simulink model "uav_full_control"  (R2023a)
settings: Solver=FixedStepAuto  StartTime=0.0  StopTime=20  FixedStep=1e-3
undefined symbols (not defined in the file or in its folder): b, c_1, c_2, c_3, c_4, c_5, c_6, c_7, c_8, c_psi, C_SMC, c_z, d, D_rot, D_transl, eps1, eps2, eps3, eps4, eta1, eta2, eta3, eta4, eulerlimit, g, J1, J2, J3, Jr, K, k1, k2, k3, K_lqr, k_phi, K_SMC, k_theta, L, m, Matrix_Force2angular_velocity, R
libraries: simulink x14, control_form_LagrangeSimplified x2, control_form_NL x2, control_form_NL_forces x2, control_form_LagrangeSimplified_forces x1
(part 2 of 2)

== matlab function uav_full_control/MATLAB Function5 ==
  data: x input; transf output; y input; z input; phi input; theta input; psi input; xdot input; ydot input; zdot input; zeta input; xi input; p input; q input; r input
function transf = transform_difeo_function(x,y,z,phi,theta,psi,xdot,ydot,zdot,zeta,xi,p,q,r)

% prep
m=1.88;
g=9.81;
J1=1.453e-2;
J2=1.453e-2;
J3=2.884e-2;

input1=0;
input2=0;
input3=0;
input4=0;

sphi=sin(phi);
cphi=cos(phi);
stheta=sin(theta);
ctheta=cos(theta);
spsi=sin(psi);
cpsi=cos(psi);

% model dynamics
phi_dot=p+q*(sin(phi)*tan(theta))+r*(cos(phi)*tan(theta));
theta_dot=q*cos(phi)-r*sin(phi);
psi_dot=q*sin(phi)/cos(theta)+r*cos(phi)/cos(theta);


zeta_dot=xi;
xi_dot=input1;

p_dot=(J2-J3)/J1*q*r+1/J1*input2;
q_dot=(J3-J1)/J2*r*p+1/J2*input3;
r_dot=(J1-J2)/J3*p*q+1/J3*input4;

%others
phi_d_dot=p_dot+q_dot*sphi*tan(theta)+phi_dot*q*cphi*tan(theta)+theta_dot*q*sphi/(ctheta^2)+...
r_dot*cphi*tan(theta)-phi_dot*r*sphi*tan(theta)+theta_dot*r*cphi/(ctheta^2);

theta_d_dot=q_dot*cphi-phi_dot*q*sphi-r_dot*sphi-r*phi_dot*cphi;

psi_d_dot=q_dot*sphi/ctheta+q/(ctheta^2)*(phi_dot*cphi*ctheta+theta_dot*sphi*stheta)+...
r_dot*cphi/ctheta+r/(ctheta^2)*(-phi_dot*sphi*ctheta+theta_dot*cphi*stheta);

%%%--------------------------------------------------------------------------------------

%x

Cx=cphi*stheta*cpsi+sphi*spsi;

Cx_dot=-phi_dot*sphi*stheta*cpsi+theta_dot*cphi*ctheta*cpsi-psi_dot*cphi*stheta*spsi...
+phi_dot*cphi*spsi+psi_dot*sphi*cpsi;

Cx_d_dot=psi_d_dot*(-sphi*stheta*cpsi+cphi*spsi)+theta_d_dot*cphi*ctheta*cpsi...
+psi_d_dot*(-cphi*stheta*spsi+sphi*cpsi)-cphi*stheta*cpsi*(phi_dot^2+theta_dot^2+psi_dot^2)...
-2*phi_dot*theta_dot*sphi*ctheta*cpsi+2*phi_dot*psi_dot*sphi*stheta*spsi...
-2*theta_dot*psi_dot*cphi*ctheta*spsi-sphi*spsi*(phi_dot^2+psi_dot^2)+2*phi_dot*psi_dot*cphi*cpsi;

x_4dots=-1/m*(input1*Cx+2*xi*Cx_dot+zeta*Cx_d_dot); % Lf4h1(x)
LgLf3h1=-1/m*[Cx,...
    1/J1*zeta*(-sphi*stheta*cpsi+cphi*spsi),...
    1/J2*zeta*((-sphi*stheta*cpsi+cphi*spsi)*sphi*tan(theta)+cphi*ctheta*cpsi*cphi+...
    (-cphi*stheta*spsi+sphi*cpsi)*sphi/ctheta),...
    1/J3*zeta*((-sphi*stheta*cpsi+cphi*spsi)*cphi*tan(theta)-cphi*ctheta*cpsi*sphi+...
    (-cphi*stheta*spsi+sphi*cpsi)*cphi/ctheta)];

Lf0h1=x;
Lf1h1=xdot;
Lf2h1=-1/m*zeta*Cx;
Lf3h1=-1/m*(xi*Cx+zeta*Cx_dot);

%y

Cy=cphi*stheta*spsi-sphi*cpsi;

Cy_dot=-phi_dot*sphi*stheta*spsi+theta_dot*cphi*ctheta*spsi+psi_dot*cphi*stheta*cpsi...
-phi_dot*cphi*cpsi+psi_dot*sphi*spsi;

Cy_d_dot=phi_d_dot*(-sphi*stheta*spsi-cphi*cpsi)+theta_d_dot*cphi*ctheta*spsi...
+psi_d_dot*(cphi*stheta*cpsi+sphi*spsi)-cphi*stheta*spsi*(phi_dot^2+theta_dot^2+psi_dot^2)...
-2*phi_dot*theta_dot*sphi*ctheta*spsi-2*phi_dot*psi_dot*sphi*stheta*cpsi...
+2*theta_dot*psi_dot*cphi*ctheta*cpsi+sphi*cpsi*(phi_dot^2+psi_dot^2)+2*phi_dot*psi_dot*cphi*spsi;

y_4dots=-1/m*(input1*Cy+2*xi*Cy_dot+zeta*Cy_d_dot);
LgLf3h2=-1/m*[Cy,...
    1/J1*zeta*(-sphi*stheta*spsi-cphi*cpsi),...
    1/J2*zeta*((-sphi*stheta*spsi-cphi*cpsi)*sphi*tan(theta)+cphi*ctheta*spsi*cphi+...
    (cphi*stheta*cpsi+sphi*spsi)*sphi/ctheta),...
    1/J3*zeta*((-sphi*stheta*spsi-cphi*cpsi)*cphi*tan(theta)-cphi*ctheta*spsi*sphi+...
    (cphi*stheta*cpsi+sphi*spsi)*cphi/ctheta)];

Lf0h2=y;
Lf1h2=ydot;
Lf2h2=-1/m*zeta*Cy;
Lf3h2=-1/m*(xi*Cy+zeta*Cy_dot);

%z
Cz=cphi*ctheta;

Cz_dot=-phi_dot*sphi*ctheta-theta_dot*cphi*stheta;

Cz_d_dot=-phi_d_dot*sphi*ctheta-phi_dot^2*cphi*ctheta+2*phi_dot*theta_dot*sphi*stheta...
    -theta_d_dot*cphi*stheta-theta_dot^2*cphi*ctheta;

z_4dots=-1/m*(input1*Cz+2*xi*Cz_dot+zeta*Cz_d_dot);
LgLf3h3=-1/m*[Cz,...
    1/J1*zeta*(-sphi*ctheta),...
    1/J2*zeta*(-sphi*ctheta*sphi*tan(theta)-cphi*stheta*cphi),...
    1/J3*zeta*(-sphi*ctheta*cphi*tan(theta)+cphi*stheta*sphi)];

Lf0h3=z;
Lf1h3=zdot;
Lf2h3=g-1/m*zeta*Cz;
Lf3h3=-1/m*(xi*Cz+zeta*Cz_dot);
%psi
Lf0h4=psi;
Lf1h4=psi_dot;
%psi_d_dot is defined above
LgLf1h4=[0,...
    0,...
    1/J2*sphi/ctheta,...
    1/J3*cphi/ctheta];
transf=[Lf0h1,Lf1h1,Lf2h1,Lf3h1,Lf0h2,Lf1h2,Lf2h2,Lf3h2,Lf0h3,Lf1h3,Lf2h3,Lf3h3,Lf0h4,Lf1h4]';

== matlab function uav_full_control/MATLAB Function6 ==
  data: states input; v_hat input; fr_hat input; C_SMC input; k_theta input; k_phi input; K_SMC input; xref input; yref input; zref input; psiref input; u output
function u = fcn_smc(states, v_hat, fr_hat, C_SMC, k_theta, k_phi, K_SMC, xref, yref, zref, psiref)
    arguments
        states (12,1) {mustBeNumeric}
        v_hat
        fr_hat
        C_SMC 
        k_theta
        k_phi
        K_SMC
        xref (5,1)
        yref (5,1)
        zref (5,1)
        psiref (3,1)
    end

 m=1.888;
 g=9.81;
 J1=1.453e-2;
 J2=1.453e-2;
 J3=2.884e-2;

 x=states(1);
 y=states(2);
 z=states(3);
 phi=states(4);
 theta=states(5);
 psi=states(6);
 xdot=states(7);
 ydot=states(8);
 zdot=states(9);
 phidot=states(10);
 thetadot=states(11);
 psidot=states(12);

 xdesired=xref(1);
 xdesired_dot=xref(2);
 ydesired=yref(1);
 ydesired_dot=yref(2);
 zdesired=zref(1);
 zdesired_dot=zref(2);
 psidesired=psiref(1);
 psidesired_dot=psiref(2);
 xdesired_d_dot=xref(3);
 ydesired_d_dot=yref(3);
 zdesired_d_dot=zref(3);
 psidesired_d_dot=psiref(3);


 ex=x-xdesired;
 ex_dot=xdot-xdesired_dot;
 ey=y-ydesired;
 ey_dot=ydot-ydesired_dot;
 ez=z-zdesired;
 ez_dot=zdot-zdesired_dot;
 epsi=psi-psidesired;
 epsi_dot=psidot-psidesired_dot;
 
 % x_d_dot=-1/m*(cos(phi)*sin(theta)*cos(psi)+sin(phi)*sin(psi))*u1; 
 % y_d_dot=-1/m*(cos(phi)*sin(theta)*sin(psi)-sin(phi)*cos(psi))*u1;
 % 
 % x_dots_3=-1/m*(-phidot*sin(phi)*sin(theta)*cos(psi)+thetadot*cos(phi)*cos(theta)*cos(psi)-...
 %     psidot*cos(phi)*sin(theta)*sin(psi)+phidot*cos(phi)*sin(psi)+psidot*sin(phi)*cos(psi))*u1+u1dot*-1/m*(cos(phi)*sin(theta)*cos(psi)+sin(phi)*sin(psi));
 % y_dots_3=-1/m*(-phidot*sin(phi)*sin(theta)*sin(psi)+thetadot*cos(phi)*cos(theta)*sin(psi)+...
 %     psidot*cos(phi)*sin(theta)*cos(psi)-phidot*cos(phi)*cos(psi)+psidot*sin(phi)*sin(psi))*u1+u1dot*-1/m*(cos(phi)*sin(theta)*sin(psi)-sin(phi)*cos(psi));

 x_d_dot=-1/m*(cos(phi)*sin(theta)*cos(psi)+sin(phi)*sin(psi)); 
 y_d_dot=-1/m*(cos(phi)*sin(theta)*sin(psi)-sin(phi)*cos(psi));

 x_dots_3=-1/m*(-phidot*sin(phi)*sin(theta)*cos(psi)+thetadot*cos(phi)*cos(theta)*cos(psi)-...
     psidot*cos(phi)*sin(theta)*sin(psi)+phidot*cos(phi)*sin(psi)+psidot*sin(phi)*cos(psi));
 y_dots_3=-1/m*(-phidot*sin(phi)*sin(theta)*sin(psi)+thetadot*cos(phi)*cos(theta)*sin(psi)+...
     psidot*cos(phi)*sin(theta)*cos(psi)-phidot*cos(phi)*cos(psi)+psidot*sin(phi)*sin(psi));

 thetadesired=ex_dot+k_theta*ex;
 thetadesired_dot=(x_d_dot-xref(3))+k_theta*ex_dot;
 phidesired=ey_dot+k_phi*ey;
 phidesired_dot=(y_d_dot-yref(3))+k_phi*ey_dot;

 thetadesired_d_dot=(x_dots_3-xref(4))+k_theta*(x_d_dot-xdesired_d_dot);
 phidesired_d_dot=(y_dots_3-yref(4))+k_phi*(y_d_dot-ydesired_d_dot);
 %

 
 ephi=phi-phidesired;
 ephi_dot=phidot-phidesired_dot;
 etheta=theta-thetadesired;
 etheta_dot=thetadot-thetadesired_dot;

 e=[ex ey ez ephi etheta epsi]';
 e_dot=[ex_dot ey_dot ez_dot ephi_dot etheta_dot epsi_dot]';
 
 s=e_dot+K_SMC*e;

 G=[x_d_dot,0,0,0,1,0;...
     y_d_dot,0,0,0,0,1;
     -1/m*cos(phi)*cos(theta),0,0,0,0,0;
     0,1/J1,0,0,0,0;
     0,0,1/J2,0,0,0;
     0,0,0,1/J3,0,0];
 Ginv=inv(G);

 f=[0;0;g;(J2-J3)/J1*thetadot*psidot;(J3-J1)/J2*psidot*phidot;(J1-J2)/J3*phidot*thetadot];
 state_desired_d_dot=[xdesired_d_dot ydesired_d_dot zdesired_d_dot phidesired_d_dot thetadesired_d_dot psidesired_d_dot]';
% u=Ginv*(-f+v_hat-fr_hat+state_desired_d_dot-K_SMC*e_dot-diag([C_SMC(1),C_SMC(2),C_SMC(3),C_SMC(4),C_SMC(5),C_SMC(6)])*[sign(s(1)) sign(s(2)) sign(s(3)) sign(s(4)) sign(s(5)) sign(s(6))]');
u=Ginv*(-f+v_hat-fr_hat+state_desired_d_dot-K_SMC*e_dot-diag([C_SMC(1),C_SMC(2),C_SMC(3),C_SMC(4),C_SMC(5),C_SMC(6)])*[saturation_f(s(1)/0.3) saturation_f(s(2)/0.3) saturation_f(s(3)/0.3) saturation_f(s(4)/0.3) saturation_f(s(5)/0.3) saturation_f(s(6)/0.3)]');
% u=Ginv*(-f-fr_hat+state_desired_d_dot-K_SMC*e_dot-diag([C_SMC(1),C_SMC(2),C_SMC(3),C_SMC(4),C_SMC(5),C_SMC(6)])*[sign(s(1)) sign(s(2)) sign(s(3)) sign(s(4)) sign(s(5)) sign(s(6))]');


 function out=saturation_f(x) 
    if(abs(x)<=1)
        out=x;
    else
        out=x/abs(x);
    end
end
end

== matlab function uav_full_control/u1 ==
  data: states input; c_z input; eps1 input; eta1 input; u1 output; zref input
function u1 = fcn_u1(states, c_z,eps1,eta1,zref)
    arguments
        states (12,1) {mustBeNumeric}
        c_z
        eps1
        eta1
        zref (5,1) {mustBeNumeric}
    end

 m=1.888;
 g=9.81;
 J1=1.453e-2;
 J2=1.453e-2;
 J3=2.884e-2;

 x=states(1);
 y=states(2);
 z=states(3);
 phi=states(4);
 theta=states(5);
 psi=states(6);
 xdot=states(7);
 ydot=states(8);
 zdot=states(9);
 phidot=states(10);
 thetadot=states(11);
 psidot=states(12);

 zdesired=zref(1);
 zdesired_dot=zref(2);
 zdesired_d_dot=zref(3);
 
 s1=c_z*(zdesired-z)+zdesired_dot-zdot;
 u1=m/(cos(phi)*cos(theta))*(g-zdesired_d_dot-c_z*(zdesired_dot-zdot)-eps1*saturation_f(s1/0.3)-eta1*s1);

  function out=saturation_f(x) 
    if(abs(x)<=1)
        out=x;
    else
        out=x/abs(x);
    end
end
end

== matlab function uav_full_control/u2 ==
  data: states input; c_5 input; c_6 input; c_7 input; u2 output; c_8 input; eps4 input; eta4 input; c_z input; eps1 input; eta1 input; zref input; yref input; phiref input
function u2 = fcn_u2(states, c_5,c_6,c_7,c_8,eps4,eta4, c_z, eps1, eta1, zref,yref,phiref)
    arguments
        states (12,1) {mustBeNumeric}
        c_5
        c_6
        c_7
        c_8
        eps4
        eta4
        c_z
        eps1
        eta1
        zref 
        yref (5,1) {mustBeNumeric}
        phiref (3,1) {mustBeNumeric}
    end

 m=1.888;
 g=9.81;
 J1=1.453e-2;
 J2=1.453e-2;
 J3=2.884e-2;
 D_rot=diag([0.3,0.3,0.1]);

 x=states(1);
 y=states(2);
 z=states(3);
 phi=states(4);
 theta=states(5);
 psi=states(6);
 xdot=states(7);
 ydot=states(8);
 zdot=states(9);
 phidot=states(10);
 thetadot=states(11);
 psidot=states(12);
 
  %u1
 zdesired=zref(1);
 zdesired_dot=zref(2);
 zdesired_d_dot=zref(3);
 
 s1=c_z*(zdesired-z)+zdesired_dot-zdot;
 u1=m/(cos(phi)*cos(theta))*(g-zdesired_d_dot-c_z*(zdesired_dot-zdot)-eps1*saturation_f(s1/0.3)-eta1*s1);

  %u2
  ydesired=yref(1);
  ydesired_dot=yref(2);
  ydesired_d_dot=yref(3);
  phidesired=phiref(1);
  phidesired_dot=phiref(2);
  phidesired_d_dot=phiref(3);
  y_d_dot=-1/m*(cos(phi)*sin(theta)*sin(psi)-sin(phi)*cos(psi))*u1;
 
 c_5=c_5/(u1*cos(psi));
 c_6=c_6/(u1*cos(psi));

 s4=c_5*(ydesired_dot-ydot)+c_6*(ydesired-y)+c_7*(phidesired_dot-phidot)+c_8*(phidesired-phi);
 u2=J1/c_7*(phidesired_d_dot+D_rot(1,1)*phidot/J1-(J2-J3)/J1*thetadot*psidot+c_8*(phidesired_dot-phidot)+c_6*(ydesired_dot-ydot)+c_5*(ydesired_d_dot-y_d_dot)+eps4*saturation_f(s4/0.3)+eta4*s4);

 function out=saturation_f(x) 
    if(abs(x)<=1)
        out=x;
    else
        out=x/abs(x);
    end
 end
end

== matlab function uav_full_control/u3 ==
  data: states input; c_1 input; c_2 input; c_3 input; u3 output; c_4 input; eps3 input; eta3 input; c_z input; eps1 input; eta1 input; zref input; xref input; thetaref input
function u3 = fcn_u3(states, c_1,c_2,c_3,c_4,eps3,eta3,c_z, eps1, eta1, zref,xref,thetaref)
    arguments
        states (12,1) {mustBeNumeric}
        c_1
        c_2
        c_3
        c_4
        eps3
        eta3
        c_z
        eps1
        eta1
        zref
        xref (5,1) {mustBeNumeric}
        thetaref (3,1) {mustBeNumeric}
    end

 m=1.888;
 g=9.81;
 J1=1.453e-2;
 J2=1.453e-2;
 J3=2.884e-2;
 D_rot=diag([0.3,0.3,0.1]);


 x=states(1);
 y=states(2);
 z=states(3);
 phi=states(4);
 theta=states(5);
 psi=states(6);
 xdot=states(7);
 ydot=states(8);
 zdot=states(9);
 phidot=states(10);
 thetadot=states(11);
 psidot=states(12);

 %u1
 zdesired=zref(1);
 zdesired_dot=zref(2);
 zdesired_d_dot=zref(3);
 
 s1=c_z*(zdesired-z)+zdesired_dot-zdot;
 u1=m/(cos(phi)*cos(theta))*(g-zdesired_d_dot-c_z*(zdesired_dot-zdot)-eps1*saturation_f(s1/0.3)-eta1*s1);
 
 %u3
 xdesired=xref(1);
 xdesired_dot=xref(2);
 xdesired_d_dot=xref(3);
 thetadesired=thetaref(1);
 thetadesired_dot=thetaref(2);
 thetadesired_d_dot=thetaref(3);
 x_d_dot=-1/m*(cos(phi)*sin(theta)*cos(psi)+sin(phi)*sin(psi))*u1;

 c_1=c_1/(u1*cos(phi)*cos(psi));
 c_2=c_2/(u1*cos(phi)*cos(psi));

 s3=c_1*(xdesired_dot-xdot)+c_2*(xdesired-x)+c_3*(thetadesired_dot-thetadot)+c_4*(thetadesired-theta);
 u3=J2/c_3*(thetadesired_d_dot+D_rot(2,2)*thetadot/J2-(J3-J1)/J2*psidot*phidot+c_4*(thetadesired_dot-thetadot)+c_2*(xdesired_dot-xdot)+c_1*(xdesired_d_dot-x_d_dot)+eps3*saturation_f(s3/0.3)+eta3*s3);
 function out=saturation_f(x) 
    if(abs(x)<=1)
        out=x;
    else
        out=x/abs(x);
    end
end
end

== matlab function uav_full_control/u4 ==
  data: states input; c_psi input; eps2 input; eta2 input; u4 output; psiref input
function u4 = fcn_u4(states, c_psi,eps2,eta2,psiref)
    arguments
        states (12,1) {mustBeNumeric}
        c_psi
        eps2
        eta2
        psiref (3,1) {mustBeNumeric}
    end

 m=1.888;
 g=9.81;
 J1=1.453e-2;
 J2=1.453e-2;
 J3=2.884e-2;

 x=states(1);
 y=states(2);
 z=states(3);
 phi=states(4);
 theta=states(5);
 psi=states(6);
 xdot=states(7);
 ydot=states(8);
 zdot=states(9);
 phidot=states(10);
 thetadot=states(11);
 psidot=states(12);

 psidesired=psiref(1);
 psidesired_dot=psiref(2);
 psidesired_d_dot=psiref(3);
 
 s2=c_psi*(psidesired-psi)+psidesired_dot-psidot;
 u4=J3*(psidesired_d_dot-(J1-J2)/J3*phidot*thetadot+c_psi*(psidesired_dot-psidot)+eps2*sign(s2)+eta2*s2);
end

== matlab function uav_full_control/MATLAB Function1 ==
  data: x input; b output; y input; z input; phi input; theta input; psi input; xdot input; ydot input; zdot input; zeta input; xi input; p input; q input; r input
function b = b_function(x,y,z,phi,theta,psi,xdot,ydot,zdot,zeta,xi,p,q,r)

% prep
m=1.88;
g=9.81;
J1=1.453e-2;
J2=1.453e-2;
J3=2.884e-2;

input1=0;
input2=0;
input3=0;
input4=0;

sphi=sin(phi);
cphi=cos(phi);
stheta=sin(theta);
ctheta=cos(theta);
spsi=sin(psi);
cpsi=cos(psi);

% model dynamics
phi_dot=p+q*(sin(phi)*tan(theta))+r*(cos(phi)*tan(theta));
theta_dot=q*cos(phi)-r*sin(phi);
psi_dot=q*sin(phi)/cos(theta)+r*cos(phi)/cos(theta);


zeta_dot=xi;
xi_dot=input1;

p_dot=(J2-J3)/J1*q*r+1/J1*input2;
q_dot=(J3-J1)/J2*r*p+1/J2*input3;
r_dot=(J1-J2)/J3*p*q+1/J3*input4;

%others
phi_d_dot=p_dot+q_dot*sphi*tan(theta)+phi_dot*q*cphi*tan(theta)+theta_dot*q*sphi/(ctheta^2)+...
r_dot*cphi*tan(theta)-phi_dot*r*sphi*tan(theta)+theta_dot*r*cphi/(ctheta^2);

theta_d_dot=q_dot*cphi-phi_dot*q*sphi-r_dot*sphi-r*phi_dot*cphi;

psi_d_dot=q_dot*sphi/ctheta+q/(ctheta^2)*(phi_dot*cphi*ctheta+theta_dot*sphi*stheta)+...
r_dot*cphi/ctheta+r/(ctheta^2)*(-phi_dot*sphi*ctheta+theta_dot*cphi*stheta);

%%%--------------------------------------------------------------------------------------

%x

Cx=cphi*stheta*cpsi+sphi*spsi;

Cx_dot=-phi_dot*sphi*stheta*cpsi+theta_dot*cphi*ctheta*cpsi-psi_dot*cphi*stheta*spsi...
+phi_dot*cphi*spsi+psi_dot*sphi*cpsi;

Cx_d_dot=psi_d_dot*(-sphi*stheta*cpsi+cphi*spsi)+theta_d_dot*cphi*ctheta*cpsi...
+psi_d_dot*(-cphi*stheta*spsi+sphi*cpsi)-cphi*stheta*cpsi*(phi_dot^2+theta_dot^2+psi_dot^2)...
-2*phi_dot*theta_dot*sphi*ctheta*cpsi+2*phi_dot*psi_dot*sphi*stheta*spsi...
-2*theta_dot*psi_dot*cphi*ctheta*spsi-sphi*spsi*(phi_dot^2+psi_dot^2)+2*phi_dot*psi_dot*cphi*cpsi;

x_4dots=-1/m*(input1*Cx+2*xi*Cx_dot+zeta*Cx_d_dot); % Lf4h1(x)
LgLf3h1=-1/m*[Cx,...
    1/J1*zeta*(-sphi*stheta*cpsi+cphi*spsi),...
    1/J2*zeta*((-sphi*stheta*cpsi+cphi*spsi)*sphi*tan(theta)+cphi*ctheta*cpsi*cphi+...
    (-cphi*stheta*spsi+sphi*cpsi)*sphi/ctheta),...
    1/J3*zeta*((-sphi*stheta*cpsi+cphi*spsi)*cphi*tan(theta)-cphi*ctheta*cpsi*sphi+...
    (-cphi*stheta*spsi+sphi*cpsi)*cphi/ctheta)];

%y

Cy=cphi*stheta*spsi-sphi*cpsi;

Cy_dot=-phi_dot*sphi*stheta*spsi+theta_dot*cphi*ctheta*spsi+psi_dot*cphi*stheta*cpsi...
-phi_dot*cphi*cpsi+psi_dot*sphi*spsi;

Cy_d_dot=phi_d_dot*(-sphi*stheta*spsi-cphi*cpsi)+theta_d_dot*cphi*ctheta*spsi...
+psi_d_dot*(cphi*stheta*cpsi+sphi*spsi)-cphi*stheta*spsi*(phi_dot^2+theta_dot^2+psi_dot^2)...
-2*phi_dot*theta_dot*sphi*ctheta*spsi-2*phi_dot*psi_dot*sphi*stheta*cpsi...
+2*theta_dot*psi_dot*cphi*ctheta*cpsi+sphi*cpsi*(phi_dot^2+psi_dot^2)+2*phi_dot*psi_dot*cphi*spsi;

y_4dots=-1/m*(input1*Cy+2*xi*Cy_dot+zeta*Cy_d_dot);
LgLf3h2=-1/m*[Cy,...
    1/J1*zeta*(-sphi*stheta*spsi-cphi*cpsi),...
    1/J2*zeta*((-sphi*stheta*spsi-cphi*cpsi)*sphi*tan(theta)+cphi*ctheta*spsi*cphi+...
    (cphi*stheta*cpsi+sphi*spsi)*sphi/ctheta),...
    1/J3*zeta*((-sphi*stheta*spsi-cphi*cpsi)*cphi*tan(theta)-cphi*ctheta*spsi*sphi+...
    (cphi*stheta*cpsi+sphi*spsi)*cphi/ctheta)];
%z
Cz=cphi*ctheta;

Cz_dot=-phi_dot*sphi*ctheta-theta_dot*cphi*stheta;

Cz_d_dot=-phi_d_dot*sphi*ctheta-phi_dot^2*cphi*ctheta+2*phi_dot*theta_dot*sphi*stheta...
    -theta_d_dot*cphi*stheta-theta_dot^2*cphi*ctheta;

z_4dots=-1/m*(input1*Cz+2*xi*Cz_dot+zeta*Cz_d_dot);
LgLf3h3=-1/m*[Cz,...
    1/J1*zeta*(-sphi*ctheta),...
    1/J2*zeta*(-sphi*ctheta*sphi*tan(theta)-cphi*stheta*cphi),...
    1/J3*zeta*(-sphi*ctheta*cphi*tan(theta)+cphi*stheta*sphi)];

%psi

%psi_d_dot is defined above
LgLf1h4=[0,...
    0,...
    1/J2*sphi/ctheta,...
    1/J3*cphi/ctheta];
b=[x_4dots;y_4dots;z_4dots;psi_d_dot];

== matlab function uav_full_control/MATLAB Function ==
  data: x input; delta_inv output; y input; z input; phi input; theta input; psi input; xdot input; ydot input; zdot input; zeta input; xi input; p input; q input; r input
function delta_inv = delta_inv_function(x,y,z,phi,theta,psi,xdot,ydot,zdot,zeta,xi,p,q,r)

% prep
m=1.88;
g=9.81;
J1=1.453e-2;
J2=1.453e-2;
J3=2.884e-2;

input1=0;
input2=0;
input3=0;
input4=0;

sphi=sin(phi);
cphi=cos(phi);
stheta=sin(theta);
ctheta=cos(theta);
spsi=sin(psi);
cpsi=cos(psi);

% model dynamics
phi_dot=p+q*(sin(phi)*tan(theta))+r*(cos(phi)*tan(theta));
theta_dot=q*cos(phi)-r*sin(phi);
psi_dot=q*sin(phi)/cos(theta)+r*cos(phi)/cos(theta);


zeta_dot=xi;
xi_dot=input1;

p_dot=(J2-J3)/J1*q*r+1/J1*input2;
q_dot=(J3-J1)/J2*r*p+1/J2*input3;
r_dot=(J1-J2)/J3*p*q+1/J3*input4;

%others
phi_d_dot=p_dot+q_dot*sphi*tan(theta)+phi_dot*q*cphi*tan(theta)+theta_dot*q*sphi/(ctheta^2)+...
r_dot*cphi*tan(theta)-phi_dot*r*sphi*tan(theta)+theta_dot*r*cphi/(ctheta^2);

theta_d_dot=q_dot*cphi-phi_dot*q*sphi-r_dot*sphi-r*phi_dot*cphi;

psi_d_dot=q_dot*sphi/ctheta+q/(ctheta^2)*(phi_dot*cphi*ctheta+theta_dot*sphi*stheta)+...
r_dot*cphi/ctheta+r/(ctheta^2)*(-phi_dot*sphi*ctheta+theta_dot*cphi*stheta);

%%%--------------------------------------------------------------------------------------

%x

Cx=cphi*stheta*cpsi+sphi*spsi;

Cx_dot=-phi_dot*sphi*stheta*cpsi+theta_dot*cphi*ctheta*cpsi-psi_dot*cphi*stheta*spsi...
+phi_dot*cphi*spsi+psi_dot*sphi*cpsi;

Cx_d_dot=psi_d_dot*(-sphi*stheta*cpsi+cphi*spsi)+theta_d_dot*cphi*ctheta*cpsi...
+psi_d_dot*(-cphi*stheta*spsi+sphi*cpsi)-cphi*stheta*cpsi*(phi_dot^2+theta_dot^2+psi_dot^2)...
-2*phi_dot*theta_dot*sphi*ctheta*cpsi+2*phi_dot*psi_dot*sphi*stheta*spsi...
-2*theta_dot*psi_dot*cphi*ctheta*spsi-sphi*spsi*(phi_dot^2+psi_dot^2)+2*phi_dot*psi_dot*cphi*cpsi;

x_4dots=-1/m*(input1*Cx+2*xi*Cx_dot+zeta*Cx_d_dot); % Lf4h1(x)
LgLf3h1=-1/m*[Cx,...
    1/J1*zeta*(-sphi*stheta*cpsi+cphi*spsi),...
    1/J2*zeta*((-sphi*stheta*cpsi+cphi*spsi)*sphi*tan(theta)+cphi*ctheta*cpsi*cphi+...
    (-cphi*stheta*spsi+sphi*cpsi)*sphi/ctheta),...
    1/J3*zeta*((-sphi*stheta*cpsi+cphi*spsi)*cphi*tan(theta)-cphi*ctheta*cpsi*sphi+...
    (-cphi*stheta*spsi+sphi*cpsi)*cphi/ctheta)];

%y

Cy=cphi*stheta*spsi-sphi*cpsi;

Cy_dot=-phi_dot*sphi*stheta*spsi+theta_dot*cphi*ctheta*spsi+psi_dot*cphi*stheta*cpsi...
-phi_dot*cphi*cpsi+psi_dot*sphi*spsi;

Cy_d_dot=phi_d_dot*(-sphi*stheta*spsi-cphi*cpsi)+theta_d_dot*cphi*ctheta*spsi...
+psi_d_dot*(cphi*stheta*cpsi+sphi*spsi)-cphi*stheta*spsi*(phi_dot^2+theta_dot^2+psi_dot^2)...
-2*phi_dot*theta_dot*sphi*ctheta*spsi-2*phi_dot*psi_dot*sphi*stheta*cpsi...
+2*theta_dot*psi_dot*cphi*ctheta*cpsi+sphi*cpsi*(phi_dot^2+psi_dot^2)+2*phi_dot*psi_dot*cphi*spsi;

y_4dots=-1/m*(input1*Cy+2*xi*Cy_dot+zeta*Cy_d_dot);
LgLf3h2=-1/m*[Cy,...
    1/J1*zeta*(-sphi*stheta*spsi-cphi*cpsi),...
    1/J2*zeta*((-sphi*stheta*spsi-cphi*cpsi)*sphi*tan(theta)+cphi*ctheta*spsi*cphi+...
    (cphi*stheta*cpsi+sphi*spsi)*sphi/ctheta),...
    1/J3*zeta*((-sphi*stheta*spsi-cphi*cpsi)*cphi*tan(theta)-cphi*ctheta*spsi*sphi+...
    (cphi*stheta*cpsi+sphi*spsi)*cphi/ctheta)];
%z
Cz=cphi*ctheta;

Cz_dot=-phi_dot*sphi*ctheta-theta_dot*cphi*stheta;

Cz_d_dot=-phi_d_dot*sphi*ctheta-phi_dot^2*cphi*ctheta+2*phi_dot*theta_dot*sphi*stheta...
    -theta_d_dot*cphi*stheta-theta_dot^2*cphi*ctheta;

z_4dots=-1/m*(input1*Cz+2*xi*Cz_dot+zeta*Cz_d_dot);
LgLf3h3=-1/m*[Cz,...
    1/J1*zeta*(-sphi*ctheta),...
    1/J2*zeta*(-sphi*ctheta*sphi*tan(theta)-cphi*stheta*cphi),...
    1/J3*zeta*(-sphi*ctheta*cphi*tan(theta)+cphi*stheta*sphi)];

%psi

%psi_d_dot is defined above
LgLf1h4=[0,...
    0,...
    1/J2*sphi/ctheta,...
    1/J3*cphi/ctheta];
delta_inv = inv([LgLf3h1;LgLf3h2;LgLf3h3;LgLf1h4]);

== matlab function uav_full_control/MATLAB Function2 ==
  data: x input; transf output; y input; z input; phi input; theta input; psi input; xdot input; ydot input; zdot input; zeta input; xi input; p input; q input; r input
function transf = transform_difeo_function(x,y,z,phi,theta,psi,xdot,ydot,zdot,zeta,xi,p,q,r)

% prep
m=1.88;
g=9.81;
J1=1.453e-2;
J2=1.453e-2;
J3=2.884e-2;

input1=0;
input2=0;
input3=0;
input4=0;

sphi=sin(phi);
cphi=cos(phi);
stheta=sin(theta);
ctheta=cos(theta);
spsi=sin(psi);
cpsi=cos(psi);

% model dynamics
phi_dot=p+q*(sin(phi)*tan(theta))+r*(cos(phi)*tan(theta));
theta_dot=q*cos(phi)-r*sin(phi);
psi_dot=q*sin(phi)/cos(theta)+r*cos(phi)/cos(theta);


zeta_dot=xi;
xi_dot=input1;

p_dot=(J2-J3)/J1*q*r+1/J1*input2;
q_dot=(J3-J1)/J2*r*p+1/J2*input3;
r_dot=(J1-J2)/J3*p*q+1/J3*input4;

%others
phi_d_dot=p_dot+q_dot*sphi*tan(theta)+phi_dot*q*cphi*tan(theta)+theta_dot*q*sphi/(ctheta^2)+...
r_dot*cphi*tan(theta)-phi_dot*r*sphi*tan(theta)+theta_dot*r*cphi/(ctheta^2);

theta_d_dot=q_dot*cphi-phi_dot*q*sphi-r_dot*sphi-r*phi_dot*cphi;

psi_d_dot=q_dot*sphi/ctheta+q/(ctheta^2)*(phi_dot*cphi*ctheta+theta_dot*sphi*stheta)+...
r_dot*cphi/ctheta+r/(ctheta^2)*(-phi_dot*sphi*ctheta+theta_dot*cphi*stheta);

%%%--------------------------------------------------------------------------------------

%x

Cx=cphi*stheta*cpsi+sphi*spsi;

Cx_dot=-phi_dot*sphi*stheta*cpsi+theta_dot*cphi*ctheta*cpsi-psi_dot*cphi*stheta*spsi...
+phi_dot*cphi*spsi+psi_dot*sphi*cpsi;

Cx_d_dot=psi_d_dot*(-sphi*stheta*cpsi+cphi*spsi)+theta_d_dot*cphi*ctheta*cpsi...
+psi_d_dot*(-cphi*stheta*spsi+sphi*cpsi)-cphi*stheta*cpsi*(phi_dot^2+theta_dot^2+psi_dot^2)...
-2*phi_dot*theta_dot*sphi*ctheta*cpsi+2*phi_dot*psi_dot*sphi*stheta*spsi...
-2*theta_dot*psi_dot*cphi*ctheta*spsi-sphi*spsi*(phi_dot^2+psi_dot^2)+2*phi_dot*psi_dot*cphi*cpsi;

x_4dots=-1/m*(input1*Cx+2*xi*Cx_dot+zeta*Cx_d_dot); % Lf4h1(x)
LgLf3h1=-1/m*[Cx,...
    1/J1*zeta*(-sphi*stheta*cpsi+cphi*spsi),...
    1/J2*zeta*((-sphi*stheta*cpsi+cphi*spsi)*sphi*tan(theta)+cphi*ctheta*cpsi*cphi+...
    (-cphi*stheta*spsi+sphi*cpsi)*sphi/ctheta),...
    1/J3*zeta*((-sphi*stheta*cpsi+cphi*spsi)*cphi*tan(theta)-cphi*ctheta*cpsi*sphi+...
    (-cphi*stheta*spsi+sphi*cpsi)*cphi/ctheta)];

Lf0h1=x;
Lf1h1=xdot;
Lf2h1=-1/m*zeta*Cx;
Lf3h1=-1/m*(xi*Cx+zeta*Cx_dot);

%y

Cy=cphi*stheta*spsi-sphi*cpsi;

Cy_dot=-phi_dot*sphi*stheta*spsi+theta_dot*cphi*ctheta*spsi+psi_dot*cphi*stheta*cpsi...
-phi_dot*cphi*cpsi+psi_dot*sphi*spsi;

Cy_d_dot=phi_d_dot*(-sphi*stheta*spsi-cphi*cpsi)+theta_d_dot*cphi*ctheta*spsi...
+psi_d_dot*(cphi*stheta*cpsi+sphi*spsi)-cphi*stheta*spsi*(phi_dot^2+theta_dot^2+psi_dot^2)...
-2*phi_dot*theta_dot*sphi*ctheta*spsi-2*phi_dot*psi_dot*sphi*stheta*cpsi...
+2*theta_dot*psi_dot*cphi*ctheta*cpsi+sphi*cpsi*(phi_dot^2+psi_dot^2)+2*phi_dot*psi_dot*cphi*spsi;

y_4dots=-1/m*(input1*Cy+2*xi*Cy_dot+zeta*Cy_d_dot);
LgLf3h2=-1/m*[Cy,...
    1/J1*zeta*(-sphi*stheta*spsi-cphi*cpsi),...
    1/J2*zeta*((-sphi*stheta*spsi-cphi*cpsi)*sphi*tan(theta)+cphi*ctheta*spsi*cphi+...
    (cphi*stheta*cpsi+sphi*spsi)*sphi/ctheta),...
    1/J3*zeta*((-sphi*stheta*spsi-cphi*cpsi)*cphi*tan(theta)-cphi*ctheta*spsi*sphi+...
    (cphi*stheta*cpsi+sphi*spsi)*cphi/ctheta)];

Lf0h2=y;
Lf1h2=ydot;
Lf2h2=-1/m*zeta*Cy;
Lf3h2=-1/m*(xi*Cy+zeta*Cy_dot);

%z
Cz=cphi*ctheta;

Cz_dot=-phi_dot*sphi*ctheta-theta_dot*cphi*stheta;

Cz_d_dot=-phi_d_dot*sphi*ctheta-phi_dot^2*cphi*ctheta+2*phi_dot*theta_dot*sphi*stheta...
    -theta_d_dot*cphi*stheta-theta_dot^2*cphi*ctheta;

z_4dots=-1/m*(input1*Cz+2*xi*Cz_dot+zeta*Cz_d_dot);
LgLf3h3=-1/m*[Cz,...
    1/J1*zeta*(-sphi*ctheta),...
    1/J2*zeta*(-sphi*ctheta*sphi*tan(theta)-cphi*stheta*cphi),...
    1/J3*zeta*(-sphi*ctheta*cphi*tan(theta)+cphi*stheta*sphi)];

Lf0h3=z;
Lf1h3=zdot;
Lf2h3=g-1/m*zeta*Cz;
Lf3h3=-1/m*(xi*Cz+zeta*Cz_dot);
%psi
Lf0h4=psi;
Lf1h4=psi_dot;
%psi_d_dot is defined above
LgLf1h4=[0,...
    0,...
    1/J2*sphi/ctheta,...
    1/J3*cphi/ctheta];
transf=[Lf0h1,Lf1h1,Lf2h1,Lf3h1,Lf0h2,Lf1h2,Lf2h2,Lf3h2,Lf0h3,Lf1h3,Lf2h3,Lf3h3,Lf0h4,Lf1h4]';

== matlab function uav_full_control/MATLAB Function3 ==
  data: x input; delta_inv output; y input; z input; phi input; theta input; psi input; xdot input; ydot input; zdot input; zeta input; xi input; p input; q input; r input
function delta_inv = delta_inv_function(x,y,z,phi,theta,psi,xdot,ydot,zdot,zeta,xi,p,q,r)

% prep
m=1.88;
g=9.81;
J1=1.453e-2;
J2=1.453e-2;
J3=2.884e-2;

input1=0;
input2=0;
input3=0;
input4=0;

sphi=sin(phi);
cphi=cos(phi);
stheta=sin(theta);
ctheta=cos(theta);
spsi=sin(psi);
cpsi=cos(psi);

% model dynamics
phi_dot=p+q*(sin(phi)*tan(theta))+r*(cos(phi)*tan(theta));
theta_dot=q*cos(phi)-r*sin(phi);
psi_dot=q*sin(phi)/cos(theta)+r*cos(phi)/cos(theta);


zeta_dot=xi;
xi_dot=input1;

p_dot=(J2-J3)/J1*q*r+1/J1*input2;
q_dot=(J3-J1)/J2*r*p+1/J2*input3;
r_dot=(J1-J2)/J3*p*q+1/J3*input4;

%others
phi_d_dot=p_dot+q_dot*sphi*tan(theta)+phi_dot*q*cphi*tan(theta)+theta_dot*q*sphi/(ctheta^2)+...
r_dot*cphi*tan(theta)-phi_dot*r*sphi*tan(theta)+theta_dot*r*cphi/(ctheta^2);

theta_d_dot=q_dot*cphi-phi_dot*q*sphi-r_dot*sphi-r*phi_dot*cphi;

psi_d_dot=q_dot*sphi/ctheta+q/(ctheta^2)*(phi_dot*cphi*ctheta+theta_dot*sphi*stheta)+...
r_dot*cphi/ctheta+r/(ctheta^2)*(-phi_dot*sphi*ctheta+theta_dot*cphi*stheta);

%%%--------------------------------------------------------------------------------------

%x

Cx=cphi*stheta*cpsi+sphi*spsi;

Cx_dot=-phi_dot*sphi*stheta*cpsi+theta_dot*cphi*ctheta*cpsi-psi_dot*cphi*stheta*spsi...
+phi_dot*cphi*spsi+psi_dot*sphi*cpsi;

Cx_d_dot=psi_d_dot*(-sphi*stheta*cpsi+cphi*spsi)+theta_d_dot*cphi*ctheta*cpsi...
+psi_d_dot*(-cphi*stheta*spsi+sphi*cpsi)-cphi*stheta*cpsi*(phi_dot^2+theta_dot^2+psi_dot^2)...
-2*phi_dot*theta_dot*sphi*ctheta*cpsi+2*phi_dot*psi_dot*sphi*stheta*spsi...
-2*theta_dot*psi_dot*cphi*ctheta*spsi-sphi*spsi*(phi_dot^2+psi_dot^2)+2*phi_dot*psi_dot*cphi*cpsi;

x_4dots=-1/m*(input1*Cx+2*xi*Cx_dot+zeta*Cx_d_dot); % Lf4h1(x)
LgLf3h1=-1/m*[Cx,...
    1/J1*zeta*(-sphi*stheta*cpsi+cphi*spsi),...
    1/J2*zeta*((-sphi*stheta*cpsi+cphi*spsi)*sphi*tan(theta)+cphi*ctheta*cpsi*cphi+...
    (-cphi*stheta*spsi+sphi*cpsi)*sphi/ctheta),...
    1/J3*zeta*((-sphi*stheta*cpsi+cphi*spsi)*cphi*tan(theta)-cphi*ctheta*cpsi*sphi+...
    (-cphi*stheta*spsi+sphi*cpsi)*cphi/ctheta)];

%y

Cy=cphi*stheta*spsi-sphi*cpsi;

Cy_dot=-phi_dot*sphi*stheta*spsi+theta_dot*cphi*ctheta*spsi+psi_dot*cphi*stheta*cpsi...
-phi_dot*cphi*cpsi+psi_dot*sphi*spsi;

Cy_d_dot=phi_d_dot*(-sphi*stheta*spsi-cphi*cpsi)+theta_d_dot*cphi*ctheta*spsi...
+psi_d_dot*(cphi*stheta*cpsi+sphi*spsi)-cphi*stheta*spsi*(phi_dot^2+theta_dot^2+psi_dot^2)...
-2*phi_dot*theta_dot*sphi*ctheta*spsi-2*phi_dot*psi_dot*sphi*stheta*cpsi...
+2*theta_dot*psi_dot*cphi*ctheta*cpsi+sphi*cpsi*(phi_dot^2+psi_dot^2)+2*phi_dot*psi_dot*cphi*spsi;

y_4dots=-1/m*(input1*Cy+2*xi*Cy_dot+zeta*Cy_d_dot);
LgLf3h2=-1/m*[Cy,...
    1/J1*zeta*(-sphi*stheta*spsi-cphi*cpsi),...
    1/J2*zeta*((-sphi*stheta*spsi-cphi*cpsi)*sphi*tan(theta)+cphi*ctheta*spsi*cphi+...
    (cphi*stheta*cpsi+sphi*spsi)*sphi/ctheta),...
    1/J3*zeta*((-sphi*stheta*spsi-cphi*cpsi)*cphi*tan(theta)-cphi*ctheta*spsi*sphi+...
    (cphi*stheta*cpsi+sphi*spsi)*cphi/ctheta)];
%z
Cz=cphi*ctheta;

Cz_dot=-phi_dot*sphi*ctheta-theta_dot*cphi*stheta;

Cz_d_dot=-phi_d_dot*sphi*ctheta-phi_dot^2*cphi*ctheta+2*phi_dot*theta_dot*sphi*stheta...
    -theta_d_dot*cphi*stheta-theta_dot^2*cphi*ctheta;

z_4dots=-1/m*(input1*Cz+2*xi*Cz_dot+zeta*Cz_d_dot);
LgLf3h3=-1/m*[Cz,...
    1/J1*zeta*(-sphi*ctheta),...
    1/J2*zeta*(-sphi*ctheta*sphi*tan(theta)-cphi*stheta*cphi),...
    1/J3*zeta*(-sphi*ctheta*cphi*tan(theta)+cphi*stheta*sphi)];

%psi

%psi_d_dot is defined above
LgLf1h4=[0,...
    0,...
    1/J2*sphi/ctheta,...
    1/J3*cphi/ctheta];
delta_inv = inv([LgLf3h1;LgLf3h2;LgLf3h3;LgLf1h4]);
